simulink model "pmsm_decoder"  (R2020b)
settings: Solver=FixedStepDiscrete  StartTime=0.0  StopTime=10  FixedStep=Ts  RelTol=1e-3
PostLoadFcn:
  | try
  | cell = struct2cell(dir(fullfile(speedgoatroot_hdlb, 'hdlsrc', 'pwm', '*.vhd')));
  | addSourceFiles = strjoin(fullfile(cell(2,:),cell(1,:)), ';');
  | hdlset_param('pwm_example_hdlc/DUT PWM and CAP', 'IPCoreAdditionalFiles', addSourceFiles);
  | end
InitFcn:
  | Ts=50e-6;     % Simulation time step
  | kp = 1e6;   % Proportional gain
  | ki =1e2;   % Integral gain
  | fsw = 5e3;     % Switching frequency
  | Vdc = 400;     % Inverter DC supply voltage
  | Rs = 0.1;     % Stator resistance
  | Ld = 2e-3;   % Inductance (d axis)
  | Lq = 2e-3;   % Inductance (q axis)
  | PM = 0.28;        % Flux linkage
  | N = 1;               % Pole pairs
undefined symbols (not defined in the file): DiscIntNeverNeededParam
libraries: powerlib x9, powerlib_meascontrol x4, eeGeneralControl x3, simulink x3, quadrature_cpulib x2, quadrature_fpgalib x2, mcbcontrolslib x1, pwm_fpgalib x1, pwm_cpulib x1, mcbplantlib x1
settings Model: ModifiedByFormat=Speedgoat GmbH  SimulationMode=external  Creator=Speedgoat GmbH  LastModifiedBy=Speedgoat GmbH
settings SolverCC: ConcurrentTasks=on  PositivePriorityOrder=on
settings DataIOCC: LimitDataPoints=on  SaveFormat=Array  ReturnWorkspaceOutputs=off
settings OptimizationCC: BlockReduction=off  ConditionallyExecuteInputs=off  DefaultParameterBehavior=Inlined  OptimizeBlockIOStorage=off
settings DebuggingCC: AlgebraicLoopMsg=error  UnderspecifiedInitializationDetection=Classic  MergeDetectMultiDrivingBlocksExec=none  SolverPrmCheckMsg=warning  InheritedTsInSrcMsg=none  SingleTaskRateTransMsg=error  TasksWithSamePriorityMsg=none  ParameterPrecisionLossMsg=none  PregeneratedLibrarySubsystemCodeDiagnostic=none  SFUnexpectedBacktrackingDiag=warning  SFNoUnconditionalDefaultTransitionDiag=warning  SFExecutionAtInitializationDiag=none  ArithmeticOperatorsInVariantConditions=warning
settings HardwareCC: ProdBitPerPointer=32  ProdBitPerSizeT=32  ProdBitPerPtrDiffT=32  ProdLargestAtomicFloat=None  ProdIntDivRoundTo=Undefined  ProdEndianess=Unspecified  ProdWordSize=32  ProdHWDeviceType=ASIC/FPGA->ASIC/FPGA  TargetBitPerPointer=64  TargetBitPerSizeT=64  TargetBitPerPtrDiffT=64  TargetLongLongMode=on  TargetIntDivRoundTo=Zero  TargetEndianess=LittleEndian  TargetWordSize=64  TargetHWDeviceType=Custom Processor->MATLAB Host Computer  ProdEqTarget=off
settings ModelReferenceCC: PropagateSignalLabelsOutOfModel=off
settings SFSimCC: SimUseLocalCustomCode=off  CustomCodeUndefinedFunction=UseInterfaceOnly
settings RTWCC: RTWUseLocalCustomCode=off  Toolchain=Simulink Real-Time Toolchain  BuildConfiguration=Faster Runs
settings CodeAppCC: StateflowObjectComments=on
settings ConfigComp: CovMetricSettings=dw  CovSaveCumulativeToWorkspaceVar=on  CovSaveSingleToWorkspaceVar=on  CovExternalEMLEnable=off

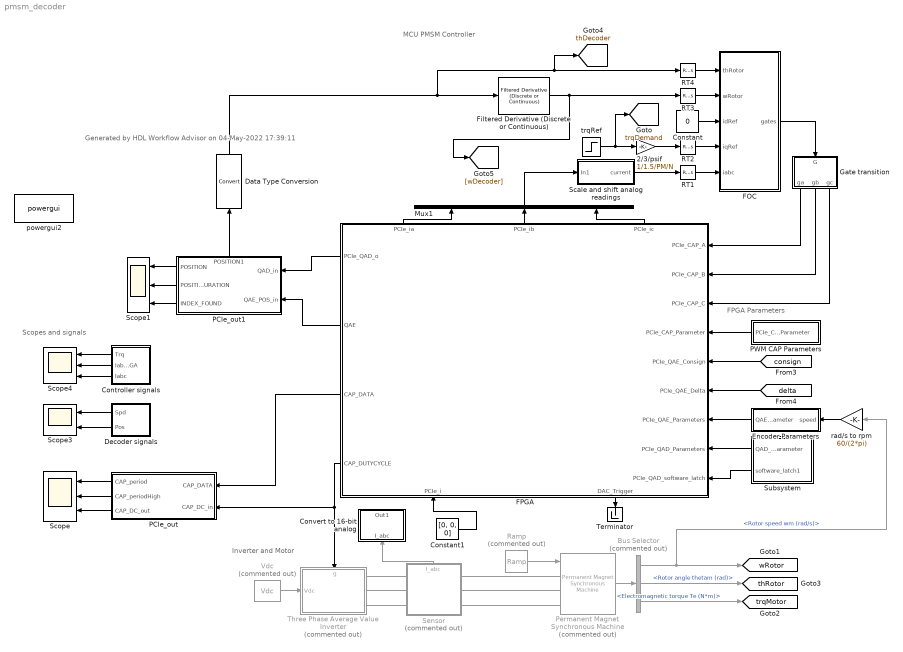
== system pmsm_decoder ==
  note: Inverter and Motor
  note: FPGA Parameters
  note: Scopes and signals
  note: MCU PMSM Controller
  note: Generated by HDL Workflow Advisor on 04-May-2022 17:39:11
  2/3/psif : Gain  Gain=1/1.5/PM/N  SaturateOnIntegerOverflow=on  OutDataTypeStr=Inherit: Same as input  ParamDataTypeStr=Inherit: Same as input
  Bus Selector : BusSelector  Commented=on  OutputSignals=Rotor speed wm (rad/s),Rotor angle thetam (rad),Electromagnetic torque Te (N*m)
  Constant : Constant  Value=0  SampleTime=-1
  Constant1 : Constant  Value=[0, 0, 0]  OutDataTypeStr=int16  SampleTime=-1
  Controller signals : Subsystem
  Convert to 16-bit analog : Subsystem
  Data Type Conversion : DataTypeConversion
  Decoder signals : Subsystem
  Encoder Parameters : Subsystem
  FOC : Subsystem
  FPGA : Subsystem
      settings: PortSchema="{\"entries\":[{\"content\":{\"sides\":[{\"content\":{\"connectorIds\":[\"Out5\",\"Out6\",\"Out7\",\"Out8\"]},\"type\":\"ConnectorPlacement.EquallySpacedRectSide\",\"uuid\":\"34ddc533-e92e-4f84-ab54-56ee31c34ed5\"},{\"content\":{\"connectorIds\":[\"In2\",\"In3\",\"In4\",\"In5\",\"In6\",\"In7\",\"In8\",\"In9\",\"In10\"],\"side\":\"RIGHT\"},\"type\":\"ConnectorPlacement.EquallySpacedRectSide\",\"uuid\":\"fc43732f-8b85-47c9-af73-b87840a05fb5\"},{\"content\":{\"connectorIds\":[\"Out2\",\"Out3\",\"Out4\"],\"side\":\"TOP\"},\"type\":\"ConnectorPlacement.EquallySpacedRectSide\",\"uuid\":\"bf663b9c-33b6-4726-afdb-56df835214b8\"},{\"content\":{\"connectorIds\":[\"In1\",\"Out1\"],\"side\":\"BOTTOM\"},\"type\":\"ConnectorPlacement.EquallySpacedRectSide\",\"uuid\":\"04fbffa8-14ef-4425-a219-a420a37a7cbf\"},{\"content\":{\"connectorIds\":[],\"side\":\"HIDDEN\"},\"type\":\"ConnectorPlacement.EquallySpacedRectSide\",\"uuid\":\"ed9b2637-afe7-435a-b994-99eac90c9c32\"}]},\"type\":\"ConnectorPlacement.EquallySpacedConnector\",\"uuid\":\"b4b9272a-3f4d-4e79-a573-4a3ad4933ba9\"}],\"packageUris\":[\"http://schema.mathworks.com/mf0/Connector/R2020b\"],\"version\":\"1.0\"}"
  Filtered Derivative (Discrete or Continuous) : eeGeneralControl/Filtered Derivative (Discrete or Continuous)  K=1  T=0.001  B=inf  A=-inf  minRatio=10  init_option=Inherited from block input  x0=0  Ts=-1
      settings: SourceProductBaseCode=PS
  Gate transition : Subsystem
  Mux1 : Mux  Inputs=3
  PCIe_out : Subsystem
  PCIe_out1 : Subsystem
      settings: PortSchema="{\"entries\":[{\"content\":{\"sides\":[{\"content\":{\"connectorIds\":[\"In1\",\"In2\"]},\"type\":\"ConnectorPlacement.EquallySpacedRectSide\",\"uuid\":\"af69b108-ebc1-4eba-857b-579d7c2071b1\"},{\"content\":{\"connectorIds\":[\"Out1\",\"Out2\",\"Out3\"],\"side\":\"RIGHT\"},\"type\":\"ConnectorPlacement.EquallySpacedRectSide\",\"uuid\":\"109121c9-5293-4b78-b0df-8505743611a0\"},{\"content\":{\"connectorIds\":[\"Out4\"],\"side\":\"TOP\"},\"type\":\"ConnectorPlacement.EquallySpacedRectSide\",\"uuid\":\"7680958f-0bbc-4169-a54e-ff3c19fd2e64\"},{\"content\":{\"connectorIds\":[],\"side\":\"HIDDEN\"},\"type\":\"ConnectorPlacement.EquallySpacedRectSide\",\"uuid\":\"af8ad87e-ac41-49e8-9442-a6b24975ced8\"}]},\"type\":\"ConnectorPlacement.EquallySpacedConnector\",\"uuid\":\"27b07649-0e95-47d8-9bc5-7790ead06fb5\"}],\"packageUris\":[\"http://schema.mathworks.com/mf0/Connector/R2020b\"],\"version\":\"1.0\"}"
  PWM CAP Parameters : Subsystem
  Permanent Magnet Synchronous Machine : powerlib/Machines/Permanent Magnet Synchronous Machine  Commented=on  NbPhases=3  FluxDistribution=Sinusoidal  RotorType=Salient-pole  MechanicalLoad=Speed w  PresetModel=No  ShowDetailedParameters=on  MeasurementBus=off  Resistance=Rs  Inductance=8.5e-3  dqInductances=[Ld Lq]  La=0.000395  MachineConstant=Flux linkage established by magnets (V.s)  Flux=PM  VoltageCst=50.7864  TorqueCst=0.42  Flat=120  Mechanical=[0.0027 0.0004924 1 0]  PolePairs=N  InitialConditions=[0,0, 0,0]  InitialConditions5ph=[0 0 0 0 0 0]  RefAngle=Aligned with phase A axis (original Park)  IterativeDiscreteModel=Trapezoidal non iterative  TsBlock=-1  TsPowergui=0
  RT{1..4} (4 alike) : RateTransition  OutPortSampleTimeOpt=Inherit  OutPortSampleTime=Ts
  Ramp : simulink/Sources/Ramp  Commented=on  slope=100/2/60*2*pi  start=0  InitialOutput=0
  Scale and shift analog readings : Subsystem
  Scope : Scope  NumInputPorts=3
  Scope1 : Scope  NumInputPorts=3
  Scope3 : Scope  NumInputPorts=2
  Scope4 : Scope  NumInputPorts=3
  Sensor : Subsystem  Commented=on
      settings: PortSchema="{\"entries\":[{\"content\":{\"sides\":[{\"content\":{\"connectorIds\":[\"LConn1\",\"LConn2\",\"LConn3\"]},\"type\":\"ConnectorPlacement.EquallySpacedRectSide\",\"uuid\":\"d3673cf9-f798-4f95-832a-0ee38b3b4235\"},{\"content\":{\"connectorIds\":[\"RConn1\",\"RConn2\",\"RConn3\"],\"side\":\"RIGHT\"},\"type\":\"ConnectorPlacement.EquallySpacedRectSide\",\"uuid\":\"f1c3e6c7-7356-4e8b-bcca-414f2c82a0be\"},{\"content\":{\"connectorIds\":[\"Out1\"],\"side\":\"TOP\"},\"type\":\"ConnectorPlacement.EquallySpacedRectSide\",\"uuid\":\"10e31bf8-a182-46d8-beca-1ec9bb9081e0\"},{\"content\":{\"connectorIds\":[],\"side\":\"HIDDEN\"},\"type\":\"ConnectorPlacement.EquallySpacedRectSide\",\"uuid\":\"21150a95-24d3-4ba1-92b8-5619804d049c\"}]},\"type\":\"ConnectorPlacement.EquallySpacedConnector\",\"uuid\":\"db0d9e3c-2d98-4024-a8e1-7fc9e86b9a02\"}],\"packageUris\":[\"http://schema.mathworks.com/mf0/Connector/R2020b\"],\"version\":\"1.0\"}"
  Subsystem : Subsystem
  Terminator : Terminator
  Three Phase Average Value Inverter : Subsystem  Commented=on
      settings: PortSchema="{\"entries\":[{\"content\":{\"sides\":[{\"content\":{\"connectorIds\":[\"In1\"]},\"type\":\"ConnectorPlacement.EquallySpacedRectSide\",\"uuid\":\"bfacb710-2d3a-4e7b-9063-25c8b87226b9\"},{\"content\":{\"connectorIds\":[\"RConn1\",\"RConn2\",\"RConn3\"],\"side\":\"RIGHT\"},\"type\":\"ConnectorPlacement.EquallySpacedRectSide\",\"uuid\":\"a8d38f79-eb95-4afe-ba2f-2842c1cba801\"},{\"content\":{\"connectorIds\":[\"In2\"],\"side\":\"TOP\"},\"type\":\"ConnectorPlacement.EquallySpacedRectSide\",\"uuid\":\"291d9d52-08e6-4456-8afe-095013b7df64\"},{\"content\":{\"connectorIds\":[],\"side\":\"HIDDEN\"},\"type\":\"ConnectorPlacement.EquallySpacedRectSide\",\"uuid\":\"61aa80b0-9b99-474b-ab67-e014373e5595\"}]},\"type\":\"ConnectorPlacement.EquallySpacedConnector\",\"uuid\":\"1232c420-125a-43af-99e1-be04cd6c95a4\"}],\"packageUris\":[\"http://schema.mathworks.com/mf0/Connector/R2020b\"],\"version\":\"1.0\"}"
  Vdc : Constant  Commented=on  Value=Vdc  SampleTime=Ts
  powergui2 : powerlib/powergui  Priority=1  SimulationMode=Discrete  SampleTime=Ts  frequency=60  Iterations=50  frequencyindice=0  Pbase=100e6  ErrMax=1e-4  UnitsV=kV  UnitsW=MW  buscounter=0  FunctionMessages=off  echomessages=off  EnableUseOfTLC=off  CurrentSourceSwitches=off  DisableSnubberDevices=off  DisableRonSwitches=off  DisableVfSwitches=off  DisplayEquations=off  AutomaticDiscreteSolvers=off  SolverType=Tustin/Backward Euler (TBE)  Interpol=off  ExternalGateDelay=off  methode=off  Ts=100  x0status=blocks  SPID=on  SwTol=0  HookPort=off  NonlinearTolerance=1e-4  nMaxIteration=100  ContinueOnMaxIteration=off  RestoreLinks=warning  ResistiveCurrentMeasurement=off  Frange=[0:2:500]  Ylog=off  Xlog=on  ShowGrid=off  save=off  variable=ZData  structure=0  ZoomFFT=off  StartTime=0.0  cycles=1  DisplayStyle=1  fundamental=60  FreqAxis=off  MaxFrequency=1000  frequencyindicesteady=1  RmsSteady=1  display=off
  rad/s to rpm : Gain  Gain=60/(2*pi)
  trqRef : Step  Time=0.3  After=300  SampleTime=Ts
  tag scope: thDecoder=global, thRotor=global, trqDemand=global, trqMotor=global, wRotor=global
  wires:
  Scale and shift analog readings/1(current) -> RT1/1
  Mux1/1 -> Scale and shift analog readings/1(In1)
  Gate transition/3(gc) -> FPGA/4(PCIe_CAP_C)
  Gate transition/2(gb) -> FPGA/3(PCIe_CAP_B)
  Gate transition/1(ga) -> FPGA/2(PCIe_CAP_A)
  [consign] -> FPGA/6(PCIe_QAE_Consign)
  [delta] -> FPGA/7(PCIe_QAE_Delta)
  Decoder signals/2(Pos) -> Scope3/2
  Decoder signals/1(Spd) -> Scope3/1
  FPGA/1(DAC_Trigger) -> Terminator/1
  FPGA/4(PCIe_ic) -> Mux1/3
  FPGA/2(PCIe_ia) -> Mux1/1
  FPGA/3(PCIe_ib) -> Mux1/2
  trqRef/1 -> [trqDemand], 2/3/psif/1
  RT1/1 -> FOC/5(iabc)
  RT2/1 -> FOC/4(iqRef)
  RT3/1 -> FOC/2(wRotor)
  FPGA/6(QAE) -> PCIe_out1/2(QAE_POS_in)
  rad/s to rpm/1 -> Encoder Parameters/1(speed)
  FPGA/7(CAP_DATA) -> PCIe_out/1(CAP_DATA)
  PWM CAP Parameters/1(PCIe_CAP_Parameter) -> FPGA/5(PCIe_CAP_Parameter)
  Encoder Parameters/1(QAE_parameter) -> FPGA/8(PCIe_QAE_Parameters)
  PCIe_out/1(CAP_period) -> Scope/1
  PCIe_out/2(CAP_periodHigh) -> Scope/2
  PCIe_out/3(CAP_DC_out) -> Scope/3
  2/3/psif/1 -> RT2/1
  Constant/1 -> FOC/3(idRef)
  FOC/1(gates) -> Gate transition/1(G)
  Bus Selector/3 -> [trqMotor]  "<Electromagnetic torque Te (N*m)>"
  Permanent Magnet Synchronous Machine/1 -> Bus Selector/1
  Bus Selector/1 -> rad/s to rpm/1, [wRotor]  "<Rotor speed wm (rad/s)>"
  Sensor/1(I_abc) -> Convert to 16-bit analog/1(I_abc)
  FPGA/8(CAP_DUTYCYCLE) -> PCIe_out/2(CAP_DC_in), Three Phase Average Value Inverter/2(g)
  Bus Selector/2 -> [thRotor]  "<Rotor angle thetam (rad)>"
  Vdc/1 -> Three Phase Average Value Inverter/1(Vdc)
  Ramp/1 -> Permanent Magnet Synchronous Machine/1
  Controller signals/1(Trq) -> Scope4/1
  Controller signals/2(Iabc_FPGA) -> Scope4/2
  Controller signals/3(Iabc) -> Scope4/3
  RT4/1 -> FOC/1(thRotor)
  Filtered Derivative (Discrete or Continuous)/1 -> RT3/1, [wDecoder]
  PCIe_out1/1(POSITION) -> Scope1/1
  PCIe_out1/3(INDEX_FOUND) -> Scope1/3
  PCIe_out1/2(POSITION_DURATION) -> Scope1/2
  FPGA/5(PCIe_QAD_o) -> PCIe_out1/1(QAD_in)
  PCIe_out1/4(POSITION1) -> Data Type Conversion/1
  Subsystem/1(QAD_parameter) -> FPGA/9(PCIe_QAD_Parameters)
  Subsystem/2(software_latch1) -> FPGA/10(PCIe_QAD_software_latch)
  Data Type Conversion/1 -> Filtered Derivative (Discrete or Continuous)/1, [thDecoder], RT4/1
  Constant1/1 -> FPGA/1(PCIe_i)
  connections:
  Permanent Magnet Synchronous Machine/LConn1 -- Sensor/RConn1
  Sensor/LConn2 -- Three Phase Average Value Inverter/RConn2
  Sensor/LConn1 -- Three Phase Average Value Inverter/RConn1
  Sensor/LConn3 -- Three Phase Average Value Inverter/RConn3
  Permanent Magnet Synchronous Machine/LConn3 -- Sensor/RConn3
  Permanent Magnet Synchronous Machine/LConn2 -- Sensor/RConn2

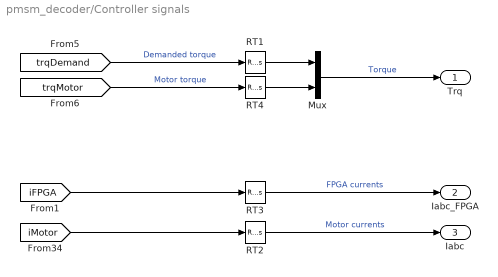
== system pmsm_decoder/Controller signals ==
  Mux : Mux  Inputs=2
  RT{1..4} (4 alike) : RateTransition  OutPortSampleTime=Ts
  Trq : Outport  VectorParamsAs1DForOutWhenUnconnected=off
  Iabc_FPGA : Outport  Port=2  VectorParamsAs1DForOutWhenUnconnected=off
  Iabc : Outport  Port=3  VectorParamsAs1DForOutWhenUnconnected=off
  wires:
  RT4/1 -> Mux/2
  [trqMotor] -> RT4/1  "Motor torque"
  Mux/1 -> Trq/1  "Torque"
  [iFPGA] -> RT3/1
  RT2/1 -> Iabc/1  "Motor currents"
  [iMotor] -> RT2/1
  RT3/1 -> Iabc_FPGA/1  "FPGA currents"
  RT1/1 -> Mux/1
  [trqDemand] -> RT1/1  "Demanded torque"

== system pmsm_decoder/Convert to 16-bit analog ==
  I_abc : Inport
  1-D Lookup Table : Lookup_n-D  NumberOfTableDimensions=1  BreakpointsForDimension1=[-2^15, 2^15-1]  Table=[0, 3.3/10*(2^15-1)]  ExtrapMethod=Clip  InternalRulePriority=Speed  RndMeth=Simplest  InputSameDT=on
  Data Type Conversion : DataTypeConversion  OutDataTypeStr=int16
  Gain : Gain  Gain=2^3
  Out1 : Outport
  wires:
  Gain/1 -> 1-D Lookup Table/1
  I_abc/1 -> Gain/1
  1-D Lookup Table/1 -> Data Type Conversion/1
  Data Type Conversion/1 -> Out1/1

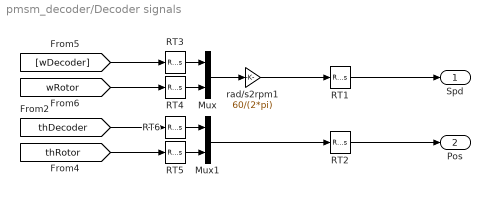
== system pmsm_decoder/Decoder signals ==
  Mux : Mux  Inputs=2
  Mux1 : Mux  Inputs=2
  RT{1..6} (6 alike) : RateTransition  OutPortSampleTime=Ts
  rad/s2rpm1 : Gain  Gain=60/(2*pi)
  Spd : Outport  VectorParamsAs1DForOutWhenUnconnected=off
  Pos : Outport  Port=2  VectorParamsAs1DForOutWhenUnconnected=off
  wires:
  RT6/1 -> Mux1/1
  RT3/1 -> Mux/1
  rad/s2rpm1/1 -> RT1/1
  RT5/1 -> Mux1/2
  RT4/1 -> Mux/2
  RT2/1 -> Pos/1
  RT1/1 -> Spd/1
  [thRotor] -> RT5/1
  [wRotor] -> RT4/1
  Mux1/1 -> RT2/1
  [thDecoder] -> RT6/1
  Mux/1 -> rad/s2rpm1/1
  [wDecoder] -> RT3/1

== system pmsm_decoder/Encoder Parameters ==
  speed : Inport
  Mux2 : Mux  Inputs=7
  Quadrature Encoder Configuration : quadrature_cpulib/Quadrature Encoder Configuration  fpgaFreq=100e6  n_channels=1  numSeg=[512]  phaseAngle=90  initPos=[0]  freeWheel=on
      settings: SourceProductName=Simulink Real-Time: Speedgoat HDL Blockset
  Step : Step  Time=0.002
  position : Constant  Value=8  SampleTime=-1
  QAE_parameter : Outport
  tag scope: consign=global, delta=global
  wires:
  Quadrature Encoder Configuration/3 -> Mux2/3
  Quadrature Encoder Configuration/9 -> [delta]
  Quadrature Encoder Configuration/1 -> Mux2/1  "position"
  Quadrature Encoder Configuration/5 -> Mux2/5
  Quadrature Encoder Configuration/6 -> Mux2/6
  Mux2/1 -> QAE_parameter/1  "QAE_parameter"
  position/1 -> Quadrature Encoder Configuration/2
  Quadrature Encoder Configuration/2 -> Mux2/2
  Quadrature Encoder Configuration/4 -> Mux2/4
  Quadrature Encoder Configuration/7 -> Mux2/7
  Step/1 -> Quadrature Encoder Configuration/1
  Quadrature Encoder Configuration/8 -> [consign]
  speed/1 -> Quadrature Encoder Configuration/3

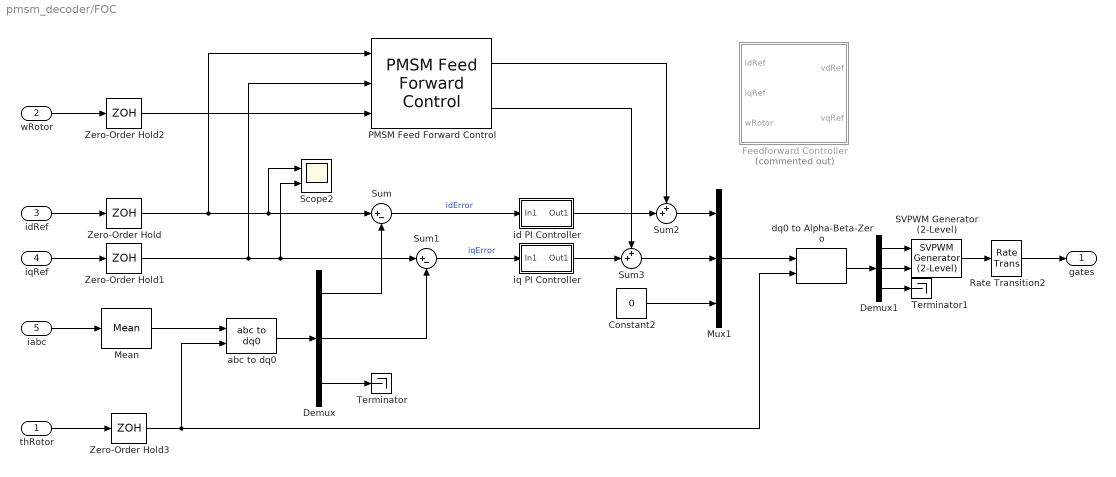
== system pmsm_decoder/FOC ==
  thRotor : Inport
  wRotor : Inport  Port=2
  idRef : Inport  Port=3
  iqRef : Inport  Port=4
  iabc : Inport  Port=5
  Constant2 : Constant  Value=0  SampleTime=-1
  Demux : Demux  Outputs=3
  Demux1 : Demux  Outputs=3
  Feedforward Controller : Subsystem  Commented=on
  Mean : powerlib_meascontrol/Measurements/Mean  Freq=fsw  Vinit=0  Ts=Ts
  Mux1 : Mux  Inputs=3
  PMSM Feed Forward Control : mcbcontrolslib/PMSM Feed Forward Control  polePairs=N  Ld=Ld  Lq=Lq  FluxPM=PM  V_dc=Vdc/sqrt(3)  Units=SI Units  V_base=24/sqrt(3)  I_base=19.3  N_base=4107
      settings: SourceProductBaseCode=MT
  Rate Transition2 : RateTransition
  SVPWM Generator (2-Level) : powerlib_meascontrol/Pulse & Signal Generators/SVPWM Generator (2-Level)  InputType=alpha-beta components  SwitchingPattern=Pattern #1  Fc=fsw  ParUref=[0.8 -30 50]  Ts=Ts
      settings: SourceProductBaseCode=PS
  Scope2 : Scope  NumInputPorts=2
  Sum : Sum  Inputs=|+-
  Sum1 : Sum  Inputs=|+-
  Sum2 : Sum  Inputs=++|
  Sum3 : Sum  Inputs=++|
  Terminator : Terminator
  Terminator1 : Terminator
  Zero-Order Hold{,1..3} (4 alike) : ZeroOrderHold  SampleTime=-1
  abc to dq0 : powerlib_meascontrol/Transformations/abc to dq0  Alignment=Aligned with phase A axis
  dq0 to Alpha-Beta-Zero : powerlib_meascontrol/Transformations/dq0 to Alpha-Beta-Zero  Alignment=Aligned with phase A axis
      settings: SourceProductBaseCode=PS
  id PI Controller : Subsystem
  iq PI Controller : Subsystem
  gates : Outport  VectorParamsAs1DForOutWhenUnconnected=off
  wires:
  Demux/3 -> Terminator/1
  iq PI Controller/1(Out1) -> Sum3/2
  Zero-Order Hold/1 -> PMSM Feed Forward Control/1, Scope2/1, Sum/1
  Demux1/1 -> SVPWM Generator (2-Level)/1
  Sum/1 -> id PI Controller/1(In1)  "idError"
  abc to dq0/1 -> Demux/1
  Zero-Order Hold1/1 -> PMSM Feed Forward Control/2, Sum1/1, Scope2/2
  Rate Transition2/1 -> gates/1
  thRotor/1 -> Zero-Order Hold3/1
  wRotor/1 -> Zero-Order Hold2/1
  Mean/1 -> abc to dq0/1
  Mux1/1 -> dq0 to Alpha-Beta-Zero/1
  Demux1/3 -> Terminator1/1
  iabc/1 -> Mean/1
  Sum1/1 -> iq PI Controller/1(In1)  "iqError"
  Demux/2 -> Sum1/2
  Sum3/1 -> Mux1/2
  Sum2/1 -> Mux1/1
  id PI Controller/1(Out1) -> Sum2/2
  SVPWM Generator (2-Level)/1 -> Rate Transition2/1
  Demux1/2 -> SVPWM Generator (2-Level)/2
  dq0 to Alpha-Beta-Zero/1 -> Demux1/1
  Demux/1 -> Sum/2
  Constant2/1 -> Mux1/3
  PMSM Feed Forward Control/1 -> Sum2/1
  PMSM Feed Forward Control/2 -> Sum3/1
  idRef/1 -> Zero-Order Hold/1
  iqRef/1 -> Zero-Order Hold1/1
  Zero-Order Hold2/1 -> PMSM Feed Forward Control/3
  Zero-Order Hold3/1 -> abc to dq0/2, dq0 to Alpha-Beta-Zero/2

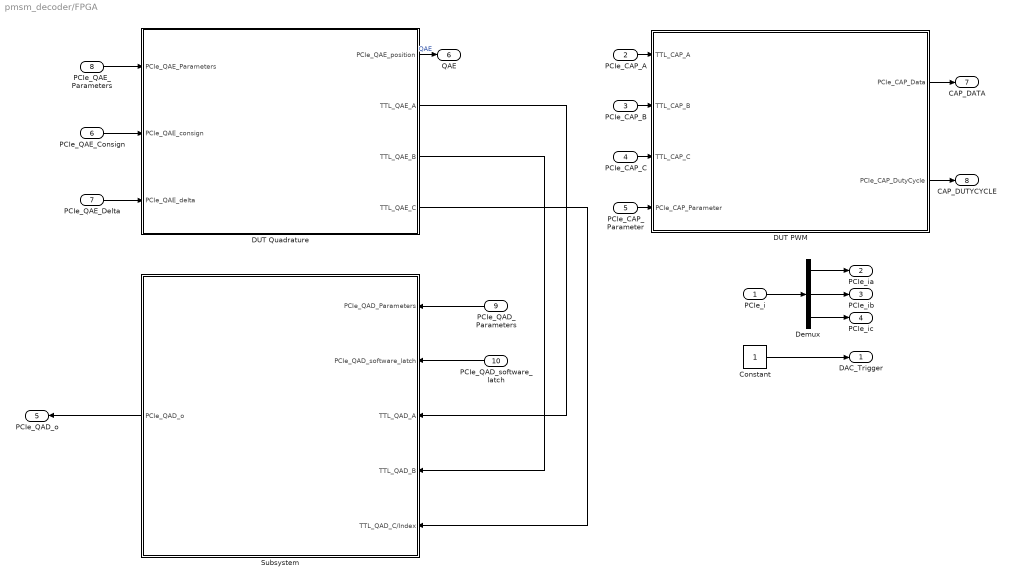
== system pmsm_decoder/FPGA ==
  PCIe_i : Inport  OutDataTypeStr=int16
  PCIe_CAP_A : Inport  Port=2
  PCIe_CAP_B : Inport  Port=3
  PCIe_CAP_C : Inport  Port=4
  PCIe_CAP_Parameter : Inport  Port=5
  PCIe_QAE_Consign : Inport  Port=6
  PCIe_QAE_Delta : Inport  Port=7
  PCIe_QAE_Parameters : Inport  Port=8
  PCIe_QAD_Parameters : Inport  Port=9
  PCIe_QAD_software_latch : Inport  Port=10
  Constant : Constant  OutDataTypeStr=boolean  SampleTime=-1
  DUT PWM : Subsystem
  DUT Quadrature : Subsystem
  Demux : Demux  Outputs=3
  Subsystem : Subsystem
  DAC_Trigger : Outport
  PCIe_ia : Outport  Port=2
  PCIe_ib : Outport  Port=3
  PCIe_ic : Outport  Port=4
  PCIe_QAD_o : Outport  Port=5  VectorParamsAs1DForOutWhenUnconnected=off
  QAE : Outport  Port=6
  CAP_DATA : Outport  Port=7
  CAP_DUTYCYCLE : Outport  Port=8
  wires:
  PCIe_QAE_Parameters/1 -> DUT Quadrature/1(PCIe_QAE_Parameters)
  PCIe_CAP_B/1 -> DUT PWM/2(TTL_CAP_B)
  PCIe_QAE_Consign/1 -> DUT Quadrature/2(PCIe_QAE_consign)
  PCIe_CAP_Parameter/1 -> DUT PWM/4(PCIe_CAP_Parameter)
  PCIe_QAE_Delta/1 -> DUT Quadrature/3(PCIe_QAE_delta)
  DUT PWM/1(PCIe_CAP_Data) -> CAP_DATA/1
  PCIe_CAP_C/1 -> DUT PWM/3(TTL_CAP_C)
  DUT Quadrature/1(PCIe_QAE_position) -> QAE/1  "QAE"
  DUT PWM/2(PCIe_CAP_DutyCycle) -> CAP_DUTYCYCLE/1
  PCIe_CAP_A/1 -> DUT PWM/1(TTL_CAP_A)
  PCIe_i/1 -> Demux/1
  Demux/1 -> PCIe_ia/1
  Demux/2 -> PCIe_ib/1
  Demux/3 -> PCIe_ic/1
  Constant/1 -> DAC_Trigger/1
  PCIe_QAD_Parameters/1 -> Subsystem/1(PCIe_QAD_Parameters)
  PCIe_QAD_software_latch/1 -> Subsystem/2(PCIe_QAD_software_latch)
  DUT Quadrature/2(TTL_QAE_A) -> Subsystem/3(TTL_QAD_A)
  DUT Quadrature/3(TTL_QAE_B) -> Subsystem/4(TTL_QAD_B)
  DUT Quadrature/4(TTL_QAE_C) -> Subsystem/5(TTL_QAD_C/Index)
  Subsystem/1(PCIe_QAD_o) -> PCIe_QAD_o/1

== system pmsm_decoder/Gate transition ==
  G : Inport
  Data Type Conversion : DataTypeConversion  OutDataTypeStr=boolean
  Demux1 : Demux  Outputs=6
  Terminator1 : Terminator
  Terminator2 : Terminator
  Terminator3 : Terminator
  ga : Outport
  gb : Outport  Port=2
  gc : Outport  Port=3
  wires:
  Demux1/5 -> gc/1
  Demux1/3 -> gb/1
  Demux1/1 -> ga/1
  Demux1/4 -> Terminator2/1
  G/1 -> Data Type Conversion/1
  Demux1/6 -> Terminator3/1
  Demux1/2 -> Terminator1/1
  Data Type Conversion/1 -> Demux1/1

== system pmsm_decoder/PCIe_out ==
  CAP_DATA : Inport
  CAP_DC_in : Inport  Port=2
  Bus Creator : BusCreator  Inputs=6
  Bus Selector : BusSelector  OutputSignals=PCIe_CAP_Period,PCIe_CAP_periodHigh
  Demux : Demux  Outputs=6
  CAP_period : Outport
  CAP_periodHigh : Outport  Port=2
  CAP_DC_out : Outport  Port=3
  wires:
  CAP_DATA/1 -> Demux/1
  Demux/5 -> Bus Creator/5  "PCIe_CAP_TOff"
  Demux/1 -> Bus Creator/1  "PCIe_CAP_Period"
  Bus Creator/1 -> Bus Selector/1
  Demux/4 -> Bus Creator/4  "PCIe_CAP_TOn"
  Demux/2 -> Bus Creator/2  "PCIe_CAP_periodHigh"
  Demux/3 -> Bus Creator/3  "PCIe_CAP_periodLow"
  Demux/6 -> Bus Creator/6  "PCIe_CAP_Data_Valid"
  Bus Selector/1 -> CAP_period/1  "<PCIe_CAP_Period>"
  Bus Selector/2 -> CAP_periodHigh/1  "<PCIe_CAP_periodHigh>"
  CAP_DC_in/1 -> CAP_DC_out/1  "CAP_DutyCycle"

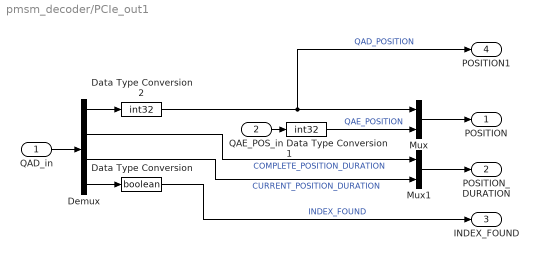
== system pmsm_decoder/PCIe_out1 ==
  QAD_in : Inport
  QAE_POS_in : Inport  Port=2
  Data Type Conversion : DataTypeConversion  OutDataTypeStr=boolean
  Data Type Conversion1 : DataTypeConversion  OutDataTypeStr=int32
  Data Type Conversion2 : DataTypeConversion  OutDataTypeStr=int32
  Demux : Demux
  Mux : Mux  Inputs=2
  Mux1 : Mux  Inputs=2
  POSITION : Outport
  POSITION_DURATION : Outport  Port=2
  INDEX_FOUND : Outport  Port=3
  POSITION1 : Outport  Port=4
  wires:
  Data Type Conversion1/1 -> Mux/2  "QAE_POSITION"
  Mux1/1 -> POSITION_DURATION/1
  Mux/1 -> POSITION/1
  Demux/2 -> Mux1/1  "COMPLETE_POSITION_DURATION"
  QAD_in/1 -> Demux/1
  Demux/3 -> Mux1/2  "CURRENT_POSITION_DURATION"
  Data Type Conversion2/1 -> POSITION1/1, Mux/1  "QAD_POSITION"
  Demux/4 -> Data Type Conversion/1
  Data Type Conversion/1 -> INDEX_FOUND/1  "INDEX_FOUND"
  Demux/1 -> Data Type Conversion2/1
  QAE_POS_in/1 -> Data Type Conversion1/1

== system pmsm_decoder/PWM CAP Parameters ==
  Data Type Conversion4 : DataTypeConversion  OutDataTypeStr=uint32
  Data Type Conversion5 : DataTypeConversion  OutDataTypeStr=uint32
  Data Type Conversion6 : DataTypeConversion  OutDataTypeStr=uint32
  Mux1 : Mux  Inputs=3
  PWM Capture Configuration : pwm_cpulib/PWM Capture Configuration  FPGA_freq=100e6  n_channels=1  captureMode=High transitions triggered  captureTimeout=0  PWM_pattern_en=off
      settings: SourceProductName=Simulink Real-Time: Speedgoat HDL Blockset
  PCIe_CAP_Parameter : Outport
  wires:
  PWM Capture Configuration/1 -> Data Type Conversion4/1
  Mux1/1 -> PCIe_CAP_Parameter/1
  PWM Capture Configuration/3 -> Data Type Conversion6/1
  Data Type Conversion4/1 -> Mux1/1
  Data Type Conversion5/1 -> Mux1/2
  Data Type Conversion6/1 -> Mux1/3
  PWM Capture Configuration/2 -> Data Type Conversion5/1

== system pmsm_decoder/Scale and shift analog readings ==
  In1 : Inport
  1-D Lookup Table : Lookup_n-D  NumberOfTableDimensions=1  BreakpointsForDimension1=[0, 3.3/10*(2^15-1)]  Table=[-2^15, 2^15-1]  ExtrapMethod=Clip  InternalRulePriority=Speed  RndMeth=Simplest  InputSameDT=on
  Data Type Conversion : DataTypeConversion  OutDataTypeStr=double
  Scale to max range : Gain  Gain=2^-3
  current : Outport
  tag scope: iFPGA=global
  wires:
  Scale to max range/1 -> [iFPGA], current/1  "current"
  In1/1 -> Data Type Conversion/1
  1-D Lookup Table/1 -> Scale to max range/1
  Data Type Conversion/1 -> 1-D Lookup Table/1

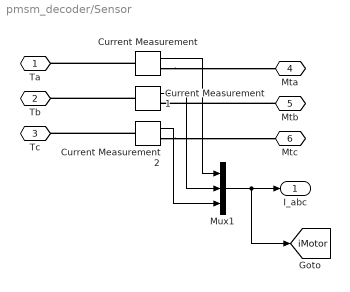
== system pmsm_decoder/Sensor ==
  Current Measurement : powerlib/Measurements/Current Measurement  PhasorSimulation=off  OutputType=Complex  PSBequivalent=0
  Current Measurement1 : powerlib/Measurements/Current Measurement  PhasorSimulation=off  OutputType=Complex  PSBequivalent=0
  Current Measurement2 : powerlib/Measurements/Current Measurement  PhasorSimulation=off  OutputType=Complex  PSBequivalent=0
  Mux1 : Mux  Inputs=3
  Ta : PMIOPort  Side=Left
  Tb : PMIOPort  Port=2  Side=Left
  Tc : PMIOPort  Port=3  Side=Left
  Mta : PMIOPort  Port=4  Side=Right
  Mtb : PMIOPort  Port=5  Side=Right
  Mtc : PMIOPort  Port=6  Side=Right
  I_abc : Outport  VectorParamsAs1DForOutWhenUnconnected=off
  tag scope: iMotor=global
  wires:
  Current Measurement1/1 -> Mux1/2
  Current Measurement/1 -> Mux1/1
  Current Measurement2/1 -> Mux1/3
  Mux1/1 -> [iMotor], I_abc/1
  connections:
  Mtb/RConn1 -- Current Measurement1/RConn1
  Current Measurement1/LConn1 -- Tb/RConn1
  Current Measurement/RConn1 -- Mta/RConn1
  Current Measurement/LConn1 -- Ta/RConn1
  Current Measurement2/LConn1 -- Tc/RConn1
  Current Measurement2/RConn1 -- Mtc/RConn1

== system pmsm_decoder/Subsystem ==
  Data Type Conversion1 : DataTypeConversion
  Mux2 : Mux  Inputs=6
  Quadrature Decoder Configuration : quadrature_cpulib/Quadrature Decoder Configuration  FPGA_freq=100e6  n_channels=1  samplingMode=4x  indexControlMode=Reset on index  latchMode=Continuous  lowerLimit=-5000  upperLimit=5000
      settings: SourceProductName=Simulink Real-Time: Speedgoat HDL Blockset
  Step : Step  Time=0.002
  Unit Delay1 : UnitDelay  SampleTime=-1  HasFrameUpgradeWarning=on
  software_latch : Constant  Value=0  SampleTime=-1
  QAD_parameter : Outport
  software_latch1 : Outport  Port=2
  wires:
  Quadrature Decoder Configuration/2 -> Mux2/2
  Unit Delay1/1 -> Quadrature Decoder Configuration/1
  Step/1 -> Data Type Conversion1/1
  Quadrature Decoder Configuration/5 -> Mux2/5
  Data Type Conversion1/1 -> Unit Delay1/1
  Quadrature Decoder Configuration/3 -> Mux2/3
  Quadrature Decoder Configuration/4 -> Mux2/4
  Quadrature Decoder Configuration/6 -> Mux2/6
  Quadrature Decoder Configuration/1 -> Mux2/1
  software_latch/1 -> Quadrature Decoder Configuration/2
  Mux2/1 -> QAD_parameter/1  "QAD_parameter"
  Quadrature Decoder Configuration/7 -> software_latch1/1

== system pmsm_decoder/Three Phase Average Value Inverter ==
  Vdc : Inport
  g : Inport  Port=2
  Average-Value Inverter : mcbplantlib/Average-Value Inverter
  Controlled Voltage Source1 : powerlib/Electrical Sources/Controlled Voltage Source  Initialize=on  Source_Type=AC  Amplitude=0  Phase=0  Frequency=0  Measurements=None
  Controlled Voltage Source3 : powerlib/Electrical Sources/Controlled Voltage Source  Initialize=on  Source_Type=AC  Amplitude=0  Phase=0  Frequency=0  Measurements=None
  Controlled Voltage Source4 : powerlib/Electrical Sources/Controlled Voltage Source  Initialize=on  Source_Type=AC  Amplitude=0  Phase=0  Frequency=0  Measurements=None
  Demux : Demux  Outputs=3
  Ground : powerlib/Elements/Ground  LConnTagsString=a
  Rate Transition : RateTransition
  A : PMIOPort  Tag=PMCPort  Side=Right
  B : PMIOPort  Tag=PMCPort  Port=2  Side=Right
  C : PMIOPort  Tag=PMCPort  Port=3  Side=Right
  wires:
  Average-Value Inverter/1 -> Rate Transition/1
  Rate Transition/1 -> Demux/1
  g/1 -> Average-Value Inverter/1
  Demux/1 -> Controlled Voltage Source3/1
  Demux/2 -> Controlled Voltage Source4/1
  Vdc/1 -> Average-Value Inverter/2
  Demux/3 -> Controlled Voltage Source1/1
  connections:
  Ground/LConn1 -- Controlled Voltage Source1/LConn1 -- Controlled Voltage Source4/LConn1 -- Controlled Voltage Source3/LConn1
  C/RConn1 -- Controlled Voltage Source1/RConn1
  B/RConn1 -- Controlled Voltage Source4/RConn1
  A/RConn1 -- Controlled Voltage Source3/RConn1

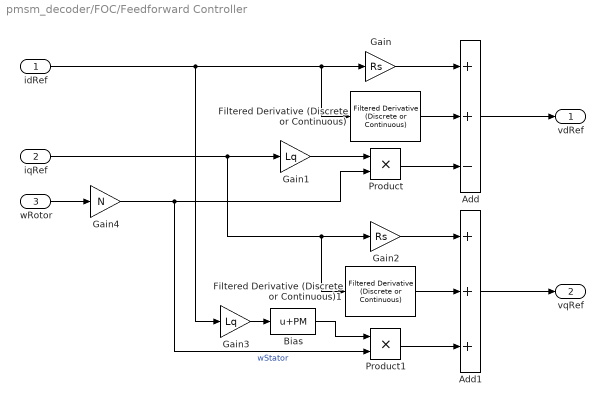
== system pmsm_decoder/FOC/Feedforward Controller ==
  idRef : Inport
  iqRef : Inport  Port=2
  wRotor : Inport  Port=3
  Add : Sum  Inputs=++-
  Add1 : Sum  Inputs=+++
  Bias : Bias  Bias=PM  SaturateOnIntegerOverflow=on
  Filtered Derivative (Discrete or Continuous) : eeGeneralControl/Filtered Derivative (Discrete or Continuous)  K=Ld  T=1e-3  B=inf  A=-inf  minRatio=10  init_option=Specify as parameter  x0=0  Ts=-1
      settings: SourceProductBaseCode=PS
  Filtered Derivative (Discrete or Continuous)1 : eeGeneralControl/Filtered Derivative (Discrete or Continuous)  K=Lq  T=1e-3  B=inf  A=-inf  minRatio=10  init_option=Specify as parameter  x0=0  Ts=-1
      settings: SourceProductBaseCode=PS
  Gain : Gain  Gain=Rs
  Gain1 : Gain  Gain=Lq
  Gain2 : Gain  Gain=Rs
  Gain3 : Gain  Gain=Lq
  Gain4 : Gain  Gain=N
  Product : Product
  Product1 : Product
  vdRef : Outport
  vqRef : Outport  Port=2
  wires:
  wRotor/1 -> Gain4/1
  Add/1 -> vdRef/1
  Gain4/1 -> Product/2, Product1/2  "wStator"
  Gain/1 -> Add/1
  idRef/1 -> Gain3/1, Filtered Derivative (Discrete or Continuous)/1, Gain/1
  Gain1/1 -> Product/1
  Product1/1 -> Add1/3
  Gain2/1 -> Add1/1
  Filtered Derivative (Discrete or Continuous)/1 -> Add/2
  iqRef/1 -> Gain2/1, Filtered Derivative (Discrete or Continuous)1/1, Gain1/1
  Filtered Derivative (Discrete or Continuous)1/1 -> Add1/2
  Bias/1 -> Product1/1
  Product/1 -> Add/3
  Gain3/1 -> Bias/1
  Add1/1 -> vqRef/1

== system pmsm_decoder/FOC/id PI Controller ==
  In1 : Inport
  Discrete-Time Integrator : DiscreteIntegrator  gainval=ki  SampleTime=-1  LimitOutput=on  UpperSaturationLimit=1  LowerSaturationLimit=-1  ICPrevOutput=DiscIntNeverNeededParam  ICPrevScaledInput=DiscIntNeverNeededParam
  Gain2 : Gain  Gain=kp  SaturateOnIntegerOverflow=on  OutDataTypeStr=Inherit: Same as input  ParamDataTypeStr=Inherit: Same as input
  Sum2 : Sum  Inputs=++|
  Out1 : Outport  VectorParamsAs1DForOutWhenUnconnected=off
  wires:
  Gain2/1 -> Sum2/2
  In1/1 -> Discrete-Time Integrator/1, Gain2/1
  Sum2/1 -> Out1/1
  Discrete-Time Integrator/1 -> Sum2/1

== system pmsm_decoder/FOC/iq PI Controller ==
  In1 : Inport
  Discrete-Time Integrator : DiscreteIntegrator  gainval=ki  SampleTime=-1  LimitOutput=on  UpperSaturationLimit=1  LowerSaturationLimit=-1  ICPrevOutput=DiscIntNeverNeededParam  ICPrevScaledInput=DiscIntNeverNeededParam
  Gain2 : Gain  Gain=kp  SaturateOnIntegerOverflow=on  OutDataTypeStr=Inherit: Same as input  ParamDataTypeStr=Inherit: Same as input
  Sum2 : Sum  Inputs=++|
  Out1 : Outport  VectorParamsAs1DForOutWhenUnconnected=off
  wires:
  Gain2/1 -> Sum2/2
  In1/1 -> Discrete-Time Integrator/1, Gain2/1
  Sum2/1 -> Out1/1
  Discrete-Time Integrator/1 -> Sum2/1

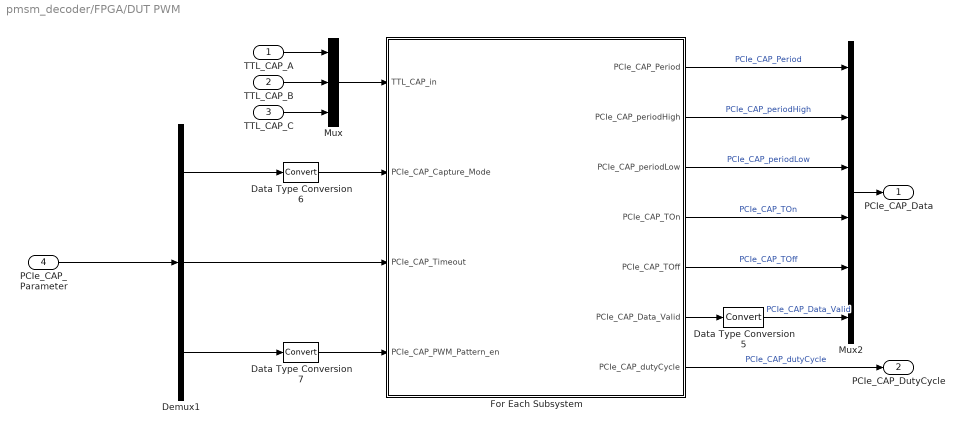
== system pmsm_decoder/FPGA/DUT PWM ==
  TTL_CAP_A : Inport
  TTL_CAP_B : Inport  Port=2
  TTL_CAP_C : Inport  Port=3
  PCIe_CAP_Parameter : Inport  Port=4
  Data Type Conversion5 : DataTypeConversion
  Data Type Conversion6 : DataTypeConversion
  Data Type Conversion7 : DataTypeConversion
  Demux1 : Demux  Outputs=3
  For Each Subsystem : Subsystem  TreatAsAtomicUnit=on
  Mux : Mux  Inputs=3
  Mux2 : Mux  Inputs=6
  PCIe_CAP_Data : Outport  VectorParamsAs1DForOutWhenUnconnected=off
  PCIe_CAP_DutyCycle : Outport  Port=2  VectorParamsAs1DForOutWhenUnconnected=off
  wires:
  Demux1/1 -> Data Type Conversion6/1
  TTL_CAP_A/1 -> Mux/1
  For Each Subsystem/7(PCIe_CAP_dutyCycle) -> PCIe_CAP_DutyCycle/1  "PCIe_CAP_dutyCycle"
  Demux1/2 -> For Each Subsystem/3(PCIe_CAP_Timeout)
  Demux1/3 -> Data Type Conversion7/1
  For Each Subsystem/6(PCIe_CAP_Data_Valid) -> Data Type Conversion5/1
  For Each Subsystem/5(PCIe_CAP_TOff) -> Mux2/5  "PCIe_CAP_TOff"
  For Each Subsystem/4(PCIe_CAP_TOn) -> Mux2/4  "PCIe_CAP_TOn"
  For Each Subsystem/3(PCIe_CAP_periodLow) -> Mux2/3  "PCIe_CAP_periodLow"
  For Each Subsystem/1(PCIe_CAP_Period) -> Mux2/1  "PCIe_CAP_Period"
  For Each Subsystem/2(PCIe_CAP_periodHigh) -> Mux2/2  "PCIe_CAP_periodHigh"
  Mux/1 -> For Each Subsystem/1(TTL_CAP_in)
  TTL_CAP_B/1 -> Mux/2
  Mux2/1 -> PCIe_CAP_Data/1
  Data Type Conversion5/1 -> Mux2/6  "PCIe_CAP_Data_Valid"
  PCIe_CAP_Parameter/1 -> Demux1/1
  Data Type Conversion6/1 -> For Each Subsystem/2(PCIe_CAP_Capture_Mode)
  Data Type Conversion7/1 -> For Each Subsystem/4(PCIe_CAP_PWM_Pattern_en)
  TTL_CAP_C/1 -> Mux/3

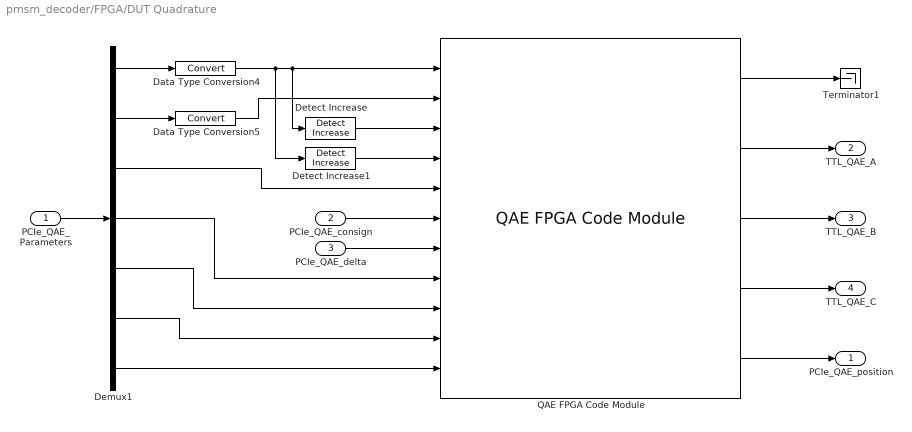
== system pmsm_decoder/FPGA/DUT Quadrature ==
  PCIe_QAE_Parameters : Inport
  PCIe_QAE_consign : Inport  Port=2  OutDataTypeStr=uint32  PortDimensions=1
  PCIe_QAE_delta : Inport  Port=3  PortDimensions=1
  Data Type Conversion4 : DataTypeConversion
  Data Type Conversion5 : DataTypeConversion
  Demux1 : Demux  Outputs=7
  Detect Increase : simulink/Logic and Bit Operations/Detect Increase  vinit=0.0  OutDataTypeStr=boolean
  Detect Increase1 : simulink/Logic and Bit Operations/Detect Increase  vinit=0.0  OutDataTypeStr=boolean
  QAE FPGA Code Module : quadrature_fpgalib/QAE FPGA Code Module  SystemSampleTime=-1  VariantActivationTime=update diagram  Latency=0  AutoFrameSizeCalculation=off
      settings: SourceProductName=Simulink Real-Time: Speedgoat Functionality Package
  Terminator1 : Terminator
  PCIe_QAE_position : Outport  VectorParamsAs1DForOutWhenUnconnected=off
  TTL_QAE_A : Outport  Port=2  VectorParamsAs1DForOutWhenUnconnected=off
  TTL_QAE_B : Outport  Port=3  VectorParamsAs1DForOutWhenUnconnected=off
  TTL_QAE_C : Outport  Port=4  VectorParamsAs1DForOutWhenUnconnected=off
  wires:
  QAE FPGA Code Module/5 -> PCIe_QAE_position/1
  Detect Increase1/1 -> QAE FPGA Code Module/4
  Detect Increase/1 -> QAE FPGA Code Module/3
  QAE FPGA Code Module/4 -> TTL_QAE_C/1
  QAE FPGA Code Module/2 -> TTL_QAE_A/1
  QAE FPGA Code Module/3 -> TTL_QAE_B/1
  PCIe_QAE_delta/1 -> QAE FPGA Code Module/7
  QAE FPGA Code Module/1 -> Terminator1/1
  PCIe_QAE_consign/1 -> QAE FPGA Code Module/6
  Demux1/1 -> Data Type Conversion4/1
  Demux1/2 -> Data Type Conversion5/1
  Demux1/3 -> QAE FPGA Code Module/5
  Demux1/4 -> QAE FPGA Code Module/8
  Demux1/5 -> QAE FPGA Code Module/9
  PCIe_QAE_Parameters/1 -> Demux1/1
  Data Type Conversion4/1 -> Detect Increase1/1, QAE FPGA Code Module/1, Detect Increase/1
  Data Type Conversion5/1 -> QAE FPGA Code Module/2
  Demux1/6 -> QAE FPGA Code Module/10
  Demux1/7 -> QAE FPGA Code Module/11

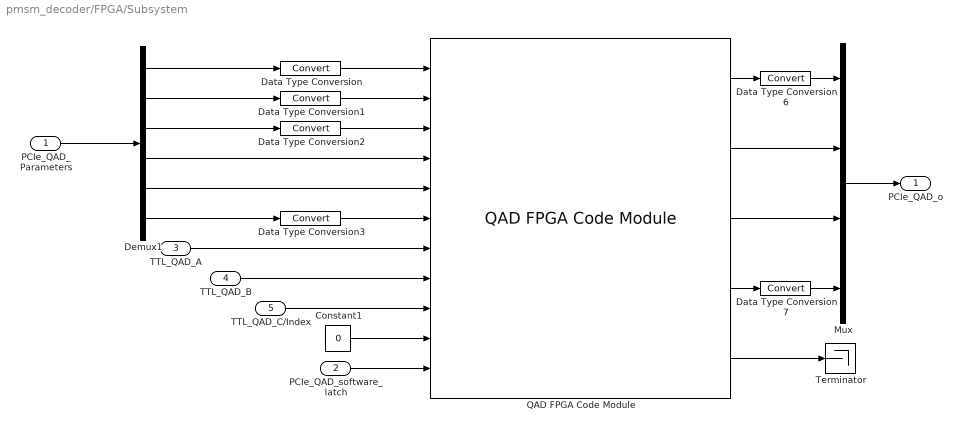
== system pmsm_decoder/FPGA/Subsystem ==
  PCIe_QAD_Parameters : Inport
  PCIe_QAD_software_latch : Inport  Port=2
  TTL_QAD_A : Inport  Port=3
  TTL_QAD_B : Inport  Port=4
  TTL_QAD_C/Index : Inport  Port=5
  Constant1 : Constant  Value=0  OutDataTypeStr=Inherit: Inherit via back propagation  SampleTime=-1
  Data Type Conversion{,1..3,6..7} (6 alike) : DataTypeConversion
  Demux1 : Demux  Outputs=6
  Mux : Mux
  QAD FPGA Code Module : quadrature_fpgalib/QAD FPGA Code Module  SystemSampleTime=-1  VariantActivationTime=update diagram  Latency=0  AutoFrameSizeCalculation=off
      settings: SourceProductName=Simulink Real-Time: Speedgoat Functionality Package
  Terminator : Terminator
  PCIe_QAD_o : Outport  VectorParamsAs1DForOutWhenUnconnected=off
  wires:
  QAD FPGA Code Module/4 -> Data Type Conversion7/1
  QAD FPGA Code Module/3 -> Mux/3
  Data Type Conversion7/1 -> Mux/4
  Demux1/4 -> QAD FPGA Code Module/4
  Demux1/6 -> Data Type Conversion3/1
  TTL_QAD_C/Index/1 -> QAD FPGA Code Module/9
  TTL_QAD_B/1 -> QAD FPGA Code Module/8
  Data Type Conversion6/1 -> Mux/1
  Data Type Conversion/1 -> QAD FPGA Code Module/1
  QAD FPGA Code Module/2 -> Mux/2
  Demux1/3 -> Data Type Conversion2/1
  Data Type Conversion2/1 -> QAD FPGA Code Module/3
  Demux1/5 -> QAD FPGA Code Module/5
  Mux/1 -> PCIe_QAD_o/1
  Data Type Conversion1/1 -> QAD FPGA Code Module/2
  PCIe_QAD_Parameters/1 -> Demux1/1
  Demux1/2 -> Data Type Conversion1/1
  Data Type Conversion3/1 -> QAD FPGA Code Module/6
  QAD FPGA Code Module/1 -> Data Type Conversion6/1
  Demux1/1 -> Data Type Conversion/1
  TTL_QAD_A/1 -> QAD FPGA Code Module/7
  Constant1/1 -> QAD FPGA Code Module/10
  QAD FPGA Code Module/5 -> Terminator/1
  PCIe_QAD_software_latch/1 -> QAD FPGA Code Module/11

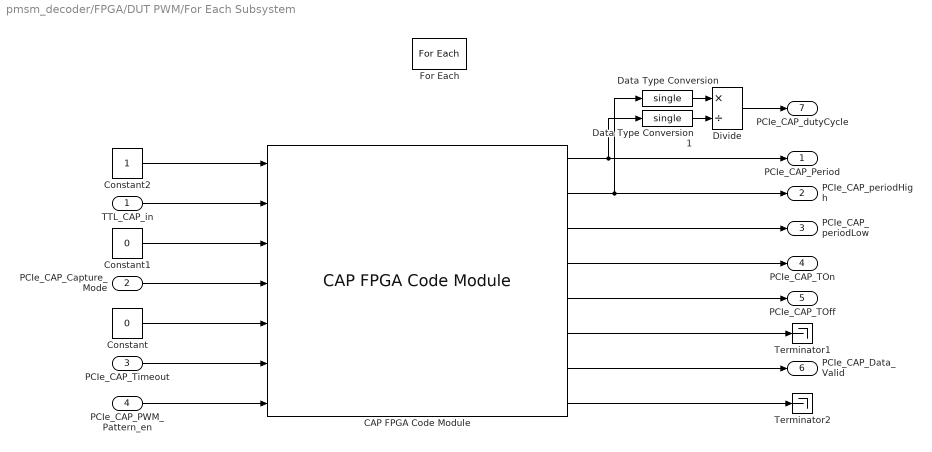
== system pmsm_decoder/FPGA/DUT PWM/For Each Subsystem ==
  TTL_CAP_in : Inport  Partition=on  PartitionDimension=1  PartitionWidth=1  PartitionOffset=0
  PCIe_CAP_Capture_Mode : Inport  Port=2
  PCIe_CAP_Timeout : Inport  Port=3
  PCIe_CAP_PWM_Pattern_en : Inport  Port=4
  CAP FPGA Code Module : pwm_fpgalib/CAP FPGA Code Module  SystemSampleTime=-1  VariantActivationTime=update diagram  Latency=0  AutoFrameSizeCalculation=off
      settings: SourceProductName=Simulink Real-Time: Speedgoat Functionality Package
  Constant : Constant  Value=0  OutDataTypeStr=Inherit: Inherit via back propagation  SampleTime=-1
  Constant1 : Constant  Value=0  OutDataTypeStr=Inherit: Inherit via back propagation  SampleTime=-1
  Constant2 : Constant  OutDataTypeStr=Inherit: Inherit via back propagation  SampleTime=-1
  Data Type Conversion : DataTypeConversion  OutMin=0  OutDataTypeStr=single
  Data Type Conversion1 : DataTypeConversion  OutMin=0  OutDataTypeStr=single  LockScale=on
  Divide : Product  Inputs=*/  RndMeth=Zero  SaturateOnIntegerOverflow=on
  For Each : ForEach  DisableCoverage=on
  Terminator1 : Terminator
  Terminator2 : Terminator
  PCIe_CAP_Period : Outport  ConcatenationDimension=2  VectorParamsAs1DForOutWhenUnconnected=off
  PCIe_CAP_periodHigh : Outport  Port=2  ConcatenationDimension=2  VectorParamsAs1DForOutWhenUnconnected=off
  PCIe_CAP_periodLow : Outport  Port=3  ConcatenationDimension=2  VectorParamsAs1DForOutWhenUnconnected=off
  PCIe_CAP_TOn : Outport  Port=4  ConcatenationDimension=2  VectorParamsAs1DForOutWhenUnconnected=off
  PCIe_CAP_TOff : Outport  Port=5  ConcatenationDimension=2  VectorParamsAs1DForOutWhenUnconnected=off
  PCIe_CAP_Data_Valid : Outport  Port=6  ConcatenationDimension=2  VectorParamsAs1DForOutWhenUnconnected=off
  PCIe_CAP_dutyCycle : Outport  Port=7  ConcatenationDimension=2  VectorParamsAs1DForOutWhenUnconnected=off
  wires:
  Data Type Conversion/1 -> Divide/1
  Divide/1 -> PCIe_CAP_dutyCycle/1
  Constant1/1 -> CAP FPGA Code Module/3
  PCIe_CAP_Capture_Mode/1 -> CAP FPGA Code Module/4
  Constant/1 -> CAP FPGA Code Module/5
  TTL_CAP_in/1 -> CAP FPGA Code Module/2
  PCIe_CAP_Timeout/1 -> CAP FPGA Code Module/6
  PCIe_CAP_PWM_Pattern_en/1 -> CAP FPGA Code Module/7
  Constant2/1 -> CAP FPGA Code Module/1
  CAP FPGA Code Module/3 -> PCIe_CAP_periodLow/1
  CAP FPGA Code Module/8 -> Terminator2/1
  CAP FPGA Code Module/5 -> PCIe_CAP_TOff/1
  CAP FPGA Code Module/6 -> Terminator1/1
  CAP FPGA Code Module/2 -> PCIe_CAP_periodHigh/1, Data Type Conversion/1
  CAP FPGA Code Module/7 -> PCIe_CAP_Data_Valid/1
  CAP FPGA Code Module/1 -> PCIe_CAP_Period/1, Data Type Conversion1/1
  CAP FPGA Code Module/4 -> PCIe_CAP_TOn/1
  Data Type Conversion1/1 -> Divide/2
